simulink model "AGTF30SysDyn_PExPIn"  (R2021b)
settings: Solver=ode4  StartTime=0.0  StopTime=MWS.In.tend  FixedStep=MWS.In.Ts  RelTol=1e-3  EnableMultiTasking=on
model workspace: external: MAT-File (data not in the file)
values from neighbouring files (symbols this model uses):
  MWS = setup_initialize(MWS,startPt,SSsolverSP)    [Setup_Simulation.m]    (also in run_AGTF30e_script.m = Setup_Simulation(inputMethod,MWS.In,filename,Mdl,SSsolverSP,)
undefined symbols (not defined in the file or in its folder): DiscIntNeverNeededParam
libraries: Lib_Solve_ModelSource_TMATS x28, Lib_Cntrl_FirstOrderSensor_TMATS x19, simulink x12, Lib_Cntrl_FirstOrderActuator_TMATS x2, Lib_Cntrl_LimitSelect_TMATS x2, Lib_Solve_OuterLoopIntegrator_TMATS x2, Lib_Cntrl_CorrectedSpeed_TMATS x1, Lib_Solve_IterNRSolverJC_TMATS x1
(part 3 of 6)

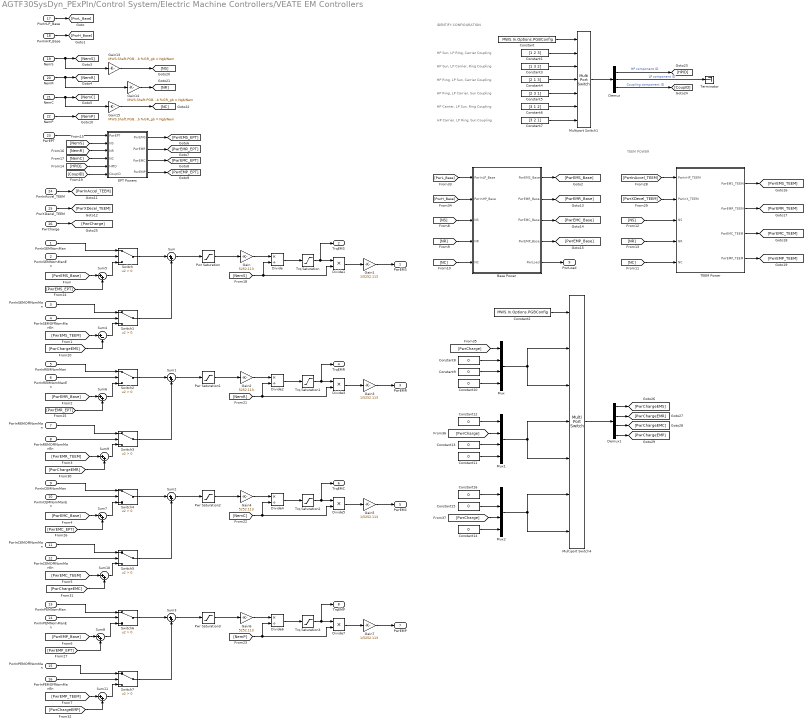
== system AGTF30SysDyn_PExPIn/Control System/Electric Machine Controllers/VEATE EM Controllers ==
  note: HP Sun, LP RIng, Carrier Coupling
  note: HP Sun, LP Carrier, Ring Coupling
  note: IDENTIFY CONFIGURATION
  note: HP Ring, LP Sun, Carrier Coupling
  note: HP Carrier, LP Sun, Ring Coupling
  note: HP Ring, LP Carrier, Sun Coupling
  note: HP Carrier, LP Ring, Sun Coupling
  note: TEEM POWER
  PwrInSEMNomMan : Inport
  PwrInSEMNomManEn : Inport  Port=2
  PwrInSEMOffNomMan : Inport  Port=3
  PwrInSEMOffNomManEn : Inport  Port=4
  PwrInREMNomMan : Inport  Port=5
  PwrInREMNomManEn : Inport  Port=6
  PwrInREMOffNomMan : Inport  Port=7
  PwrInREMOffNomManEn : Inport  Port=8
  PwrInCEMNomMan : Inport  Port=9
  PwrInCEMNomManEn : Inport  Port=10
  PwrInCEMOffNomMan : Inport  Port=11
  PwrInCEMOffNomManEn : Inport  Port=12
  PwrInPEMNomMan : Inport  Port=13
  PwrInPEMNomManEn : Inport  Port=14
  PwrInPEMOffNomMan : Inport  Port=15
  PwrInPEMOffNomManEn : Inport  Port=16
  PwrInLP_Base : Inport  Port=17
  PwrInHP_Base : Inport  Port=18
  NemS : Inport  Port=19
  NemR : Inport  Port=20
  NemC : Inport  Port=21
  NemP : Inport  Port=22
  PwrEPT : Inport  Port=23
  PwrInAccel_TEEM : Inport  Port=24
  PwrXDecel_TEEM : Inport  Port=25
  PwrCharge : Inport  Port=26
  Base Power : Subsystem
  Constant : Constant  Value=MWS.In.Options.PGBConfig
  Constant1 : Constant  Value=[1 2 3]
  Constant{8..16} (9 alike) : Constant  Value=0
  Constant2 : Constant  Value=MWS.In.Options.PGBConfig
  Constant3 : Constant  Value=[1 3 2]
  Constant4 : Constant  Value=[2 1 3]
  Constant5 : Constant  Value=[2 3 1]
  Constant6 : Constant  Value=[3 1 2]
  Constant7 : Constant  Value=[3 2 1]
  Demux : Demux  Outputs=3
  Demux1 : Demux
  Divide{,2,4,6} (4 alike) : Product  Inputs=*/
  Divide{1,3,5,7} (4 alike) : Product  Inputs=**
  EPT Powers : Subsystem
  Gain{,2,4,6} (4 alike) : Gain  Gain=5252.113
  Gain{1,3,5,7} (4 alike) : Gain  Gain=1/5252.113
  Gain13 : Gain  Gain=MWS.Shaft.PGB.Sun.GR_gb %GR_gb = Ngb/Nem
  Gain14 : Gain  Gain=MWS.Shaft.PGB.Ring.GR_gb %GR_gb = Ngb/Nem
  Gain15 : Gain  Gain=MWS.Shaft.PGB.Carrier.GR_gb %GR_gb = Ngb/Nem
  Multiport Switch1 : MultiPortSwitch  Inputs=6
  Multiport Switch4 : MultiPortSwitch  Inputs=6
  Mux : Mux
  Mux1 : Mux
  Mux2 : Mux
  Pwr Saturation : Saturate  UpperLimit=MWS.PowerSystem.EMS.PMax  LowerLimit=-MWS.PowerSystem.EMS.PMax
  Pwr Saturation1 : Saturate  UpperLimit=MWS.PowerSystem.EMR.PMax  LowerLimit=-MWS.PowerSystem.EMR.PMax
  Pwr Saturation2 : Saturate  UpperLimit=MWS.PowerSystem.EMC.PMax  LowerLimit=-MWS.PowerSystem.EMC.PMax
  Pwr Saturation3 : Saturate  UpperLimit=MWS.PowerSystem.EMP.PMax  LowerLimit=-MWS.PowerSystem.EMP.PMax
  Sum{,1..3,5..11} (11 alike) : Sum  Inputs=|++
  Sum4 : Sum  Inputs=|+-
  Switch{,1..7} (8 alike) : Switch  Criteria=u2 > Threshold
  TEEM Power : Subsystem
  Terminator : Terminator
  Trq Saturation : Saturate  UpperLimit=MWS.PowerSystem.EMS.TrqMax  LowerLimit=-MWS.PowerSystem.EMS.TrqMax
  Trq Saturation1 : Saturate  UpperLimit=MWS.PowerSystem.EMR.TrqMax  LowerLimit=-MWS.PowerSystem.EMR.TrqMax
  Trq Saturation2 : Saturate  UpperLimit=MWS.PowerSystem.EMC.TrqMax  LowerLimit=-MWS.PowerSystem.EMC.TrqMax
  Trq Saturation3 : Saturate  UpperLimit=MWS.PowerSystem.EMP.TrqMax  LowerLimit=-MWS.PowerSystem.EMP.TrqMax
  PwrEMS : Outport
  TrqEMS : Outport  Port=2
  PwrEMR : Outport  Port=3
  TrqEMR : Outport  Port=4
  PwrEMC : Outport  Port=5
  TrqEMC : Outport  Port=6
  PwrEMP : Outport  Port=7
  TrqEMP : Outport  Port=8
  PwrLoad : Outport  Port=9
  wires:
  PwrInSEMNomManEn/1 -> Switch/2
  PwrInSEMNomMan/1 -> Switch/1
  Switch/1 -> Sum/1
  Switch1/1 -> Sum/2
  PwrInSEMOffNomManEn/1 -> Switch1/2
  PwrInSEMOffNomMan/1 -> Switch1/1
  Sum/1 -> Pwr Saturation/1
  Pwr Saturation/1 -> Gain/1
  Gain/1 -> Divide/1
  [NemS] -> Divide/2, Divide1/2
  Divide/1 -> Trq Saturation/1
  Trq Saturation/1 -> Divide1/1, TrqEMS/1
  Divide1/1 -> Gain1/1
  Gain1/1 -> PwrEMS/1
  PwrInAccel_TEEM/1 -> [PwrInAccel_TEEM]
  PwrInLP_Base/1 -> [PwrL_Base]
  PwrInHP_Base/1 -> [PwrH_Base]
  [PwrEMS_Base] -> Sum5/1
  [PwrEMS_TEEM] -> Sum4/1
  Sum1/1 -> Pwr Saturation1/1
  Switch3/1 -> Sum1/2
  PwrInREMOffNomManEn/1 -> Switch3/2
  [PwrEMR_TEEM] -> Sum9/1
  [PwrEMR_Base] -> Sum6/1
  Divide3/1 -> Gain3/1
  [NemR] -> Divide2/2, Divide3/2
  Pwr Saturation1/1 -> Gain2/1
  Gain2/1 -> Divide2/1
  PwrInREMNomMan/1 -> Switch2/1
  Switch2/1 -> Sum1/1
  Divide2/1 -> Trq Saturation1/1
  Gain3/1 -> PwrEMR/1
  PwrInREMOffNomMan/1 -> Switch3/1
  Trq Saturation1/1 -> TrqEMR/1, Divide3/1
  PwrInREMNomManEn/1 -> Switch2/2
  Sum2/1 -> Pwr Saturation2/1
  Switch5/1 -> Sum2/2
  PwrInCEMOffNomManEn/1 -> Switch5/2
  [PwrEMC_TEEM] -> Sum10/1
  [PwrEMC_Base] -> Sum7/1
  Divide5/1 -> Gain5/1
  [NemC] -> Divide5/2, Divide4/2
  Pwr Saturation2/1 -> Gain4/1
  Gain4/1 -> Divide4/1
  PwrInCEMNomMan/1 -> Switch4/1
  Switch4/1 -> Sum2/1
  Divide4/1 -> Trq Saturation2/1
  Gain5/1 -> PwrEMC/1
  PwrInCEMOffNomMan/1 -> Switch5/1
  Trq Saturation2/1 -> TrqEMC/1, Divide5/1
  PwrInCEMNomManEn/1 -> Switch4/2
  Sum3/1 -> Pwr Saturation3/1
  Switch7/1 -> Sum3/2
  PwrInPEMOffNomManEn/1 -> Switch7/2
  [PwrEMP_TEEM] -> Sum11/1
  [PwrEMP_Base] -> Sum8/1
  Divide7/1 -> Gain7/1
  [NemP] -> Divide7/2, Divide6/2
  Pwr Saturation3/1 -> Gain6/1
  Gain6/1 -> Divide6/1
  PwrInPEMNomMan/1 -> Switch6/1
  Switch6/1 -> Sum3/1
  Divide6/1 -> Trq Saturation3/1
  Gain7/1 -> PwrEMP/1
  PwrInPEMOffNomMan/1 -> Switch7/1
  Trq Saturation3/1 -> TrqEMP/1, Divide7/1
  PwrInPEMNomManEn/1 -> Switch6/2
  NemS/1 -> Gain13/1, [NemS]
  NemC/1 -> Gain15/1, [NemC]
  NemP/1 -> [NemP]
  [NemC] -> EPT Powers/4(NC)
  [NemR] -> EPT Powers/3(NR)
  [NemS] -> EPT Powers/2(NS)
  PwrEPT/1 -> EPT Powers/1(PwrEPT)
  EPT Powers/1(PwrEMS) -> [PwrEMS_EPT]
  EPT Powers/2(PwrEMR) -> [PwrEMR_EPT]
  EPT Powers/3(PwrEMC) -> [PwrEMC_EPT]
  EPT Powers/4(PwrEMP) -> [PwrEMP_EPT]
  PwrXDecel_TEEM/1 -> [PwrXDecel_TEEM]
  Sum5/1 -> Switch/3
  [PwrEMS_EPT] -> Sum5/2
  Sum6/1 -> Switch2/3
  Sum7/1 -> Switch4/3
  Sum8/1 -> Switch6/3
  [PwrEMR_EPT] -> Sum6/2
  [PwrEMC_EPT] -> Sum7/2
  [PwrEMP_EPT] -> Sum8/2
  Gain13/1 -> [NS]
  Gain15/1 -> [NC]
  NemR/1 -> Gain14/1, [NemR]
  Gain14/1 -> [NR]
  Base Power/1(PwrEMS_Base) -> [PwrEMS_Base]
  Base Power/2(PwrEMR_Base) -> [PwrEMR_Base]
  Base Power/3(PwrEMC_Base) -> [PwrEMC_Base]
  Base Power/4(PwrEMP_Base) -> [PwrEMP_Base]
  [NC] -> Base Power/5(NC)
  [NR] -> Base Power/4(NR)
  [NS] -> Base Power/3(NS)
  [PwrH_Base] -> Base Power/2(PwrInHP_Base)
  [PwrL_Base] -> Base Power/1(PwrInLP_Base)
  [PwrInAccel_TEEM] -> TEEM Power/1(PwrInHP_TEEM)
  [PwrXDecel_TEEM] -> TEEM Power/2(PwrInX_TEEM)
  [NS] -> TEEM Power/3(NS)
  [NR] -> TEEM Power/4(NR)
  [NC] -> TEEM Power/5(NC)
  TEEM Power/1(PwrEMS_TEEM) -> [PwrEMS_TEEM]
  TEEM Power/2(PwrEMR_TEEM) -> [PwrEMR_TEEM]
  TEEM Power/3(PwrEMC_TEEM) -> [PwrEMC_TEEM]
  TEEM Power/4(PwrEMP_TEEM) -> [PwrEMP_TEEM]
  Demux/3 -> [CoupID]  "Coupling component ID"
  Demux/2 -> Terminator/1  "LP component ID"
  Constant5/1 -> Multiport Switch1/5
  Constant6/1 -> Multiport Switch1/6
  Multiport Switch1/1 -> Demux/1
  Constant1/1 -> Multiport Switch1/2
  Constant7/1 -> Multiport Switch1/7
  Constant/1 -> Multiport Switch1/1
  Constant3/1 -> Multiport Switch1/3
  Constant4/1 -> Multiport Switch1/4
  Demux/1 -> [HPID]  "HP component ID"
  [HPID] -> EPT Powers/5(HPID)
  [CoupID] -> EPT Powers/6(CoupID)
  PwrCharge/1 -> [PwrCharge]
  Base Power/5(PwrLoad) -> PwrLoad/1
  Sum4/1 -> Switch1/3
  [PwrChargeEMS] -> Sum4/2
  [PwrChargeEMR] -> Sum9/2
  [PwrChargeEMC] -> Sum10/2
  [PwrChargeEMP] -> Sum11/2
  Sum9/1 -> Switch3/3
  Sum10/1 -> Switch5/3
  Sum11/1 -> Switch7/3
  Constant2/1 -> Multiport Switch4/1
  Multiport Switch4/1 -> Demux1/1
  [PwrCharge] -> Mux/1
  Constant8/1 -> Mux/2
  Constant9/1 -> Mux/3
  Constant10/1 -> Mux/4
  Demux1/1 -> [PwrChargeEMS]
  Demux1/2 -> [PwrChargeEMR]
  Demux1/3 -> [PwrChargeEMC]
  Demux1/4 -> [PwrChargeEMP]
  Mux/1 -> Multiport Switch4/2, Multiport Switch4/3
  Constant11/1 -> Mux1/4
  [PwrCharge] -> Mux1/2
  Constant12/1 -> Mux1/1
  Constant13/1 -> Mux1/3
  Mux1/1 -> Multiport Switch4/5, Multiport Switch4/4
  Constant14/1 -> Mux2/4
  [PwrCharge] -> Mux2/3
  Constant15/1 -> Mux2/2
  Constant16/1 -> Mux2/1
  Mux2/1 -> Multiport Switch4/6, Multiport Switch4/7

== system AGTF30SysDyn_PExPIn/Control System/Scheduling/MaxMin Fuel Flow Calc ==
  k_Alt : Inport
  f_Alt : Inport  Port=2
  k_MN : Inport  Port=3
  f_MN : Inport  Port=4
  k_PwrInLPMx : Inport  Port=5
  f_PwrInLPMx : Inport  Port=6
  k_PwrInLPMn : Inport  Port=7
  f_PwrInLPMn : Inport  Port=8
  k_PwrInHPMx : Inport  Port=9
  f_PwrInHPMx : Inport  Port=10
  k_PwrInHPMn : Inport  Port=11
  f_PwrInHPMn : Inport  Port=12
  Wfmax Interpolation Using Prelookup : Interpolation_n-D  NumberOfTableDimensions=4  Table=MWS.Cntrl.Sched.WfMax.WfMax_array  InternalRulePriority=Speed
      settings: InputPortMap=u0,u1,u2,u3,u4,u5,u6,u7
  Wfmin Interpolation Using Prelookup : Interpolation_n-D  NumberOfTableDimensions=4  Table=MWS.Cntrl.Sched.WfMin.WfMin_array  InternalRulePriority=Speed
      settings: InputPortMap=u0,u1,u2,u3,u4,u5,u6,u7
  Wfmin : Outport  VectorParamsAs1DForOutWhenUnconnected=off
  Wfmax : Outport  Port=2  VectorParamsAs1DForOutWhenUnconnected=off
  wires:
  f_PwrInLPMn/1 -> Wfmin Interpolation Using Prelookup/6
  k_PwrInLPMn/1 -> Wfmin Interpolation Using Prelookup/5
  f_PwrInLPMx/1 -> Wfmax Interpolation Using Prelookup/6
  k_PwrInLPMx/1 -> Wfmax Interpolation Using Prelookup/5
  f_MN/1 -> Wfmax Interpolation Using Prelookup/4, Wfmin Interpolation Using Prelookup/4
  k_MN/1 -> Wfmax Interpolation Using Prelookup/3, Wfmin Interpolation Using Prelookup/3
  f_Alt/1 -> Wfmax Interpolation Using Prelookup/2, Wfmin Interpolation Using Prelookup/2
  k_Alt/1 -> Wfmax Interpolation Using Prelookup/1, Wfmin Interpolation Using Prelookup/1
  Wfmin Interpolation Using Prelookup/1 -> Wfmin/1
  Wfmax Interpolation Using Prelookup/1 -> Wfmax/1
  k_PwrInHPMx/1 -> Wfmax Interpolation Using Prelookup/7
  f_PwrInHPMx/1 -> Wfmax Interpolation Using Prelookup/8
  k_PwrInHPMn/1 -> Wfmin Interpolation Using Prelookup/7
  f_PwrInHPMn/1 -> Wfmin Interpolation Using Prelookup/8

== system AGTF30SysDyn_PExPIn/Control System/Scheduling/Power Level Lookup Determination ==
  k_Alt : Inport
  f_Alt : Inport  Port=2
  k_MN : Inport  Port=3
  f_MN : Inport  Port=4
  k_PwrInLPMn : Inport  Port=5
  f_PwrInLPMx : Inport  Port=6
  k_PwrInHPMn : Inport  Port=7
  f_PwrInHPMx : Inport  Port=8
  FnTarget : Inport  Port=9
  N1c : Inport  Port=10
  Constant1 : Constant  Value=MWS.Cntrl.SPSched.PL_vec
  Constant35 : Constant  Value=[[0:1:length(MWS.Cntrl.SPSched.PL_vec)-2],length(MWS.Cntrl.SPSched.PL_vec)-2]
  Constant36 : Constant  Value=[zeros(1,length(MWS.Cntrl.SPSched.PL_vec)-1),1]
  Fn Interpolation Using Prelookup : Interpolation_n-D  NumberOfTableDimensions=5  Table=MWS.Cntrl.Sched.Fn.Fn_array  InternalRulePriority=Speed
      settings: InputPortMap=u0,u1,u2,u3,u4,u5,u6,u7,u8,u9
  Fn Lookup Table Dynamic : simulink/Lookup Tables/Lookup Table Dynamic  LookUpMeth=Interpolation-Use End Values  OutDataType=fixdt('double')  OutScaling=[]  OutputDataTypeScalingMode=Specify via dialog  OutDataTypeStr=double  DoSatur=off
  N1c Interpolation Using Prelookup1 : Interpolation_n-D  NumberOfTableDimensions=5  Table=MWS.Cntrl.WfCntrl.Sched.N1cSP.N1cSP_array  InternalRulePriority=Speed
      settings: InputPortMap=u0,u1,u2,u3,u4,u5,u6,u7,u8,u9
  N1c Lookup Table Dynamic : simulink/Lookup Tables/Lookup Table Dynamic  LookUpMeth=Interpolation-Use End Values  OutDataType=fixdt('double')  OutScaling=[]  OutputDataTypeScalingMode=Specify via dialog  OutDataTypeStr=double  DoSatur=off
  PL Prelookup1 : PreLookup  BreakpointsData=MWS.Cntrl.SPSched.PL_vec  IndexSearchMethod=Linear search  BeginIndexSearchUsingPreviousIndexResult=on  ExtrapMethod=Linear
  PL Targ Prelookup : PreLookup  BreakpointsData=MWS.Cntrl.SPSched.PL_vec  IndexSearchMethod=Linear search  BeginIndexSearchUsingPreviousIndexResult=on  ExtrapMethod=Linear
  k_PL_Targ : Outport
  f_PL_Targ : Outport  Port=2
  k_PL : Outport  Port=3
  f_PL : Outport  Port=4
  wires:
  f_PwrInHPMx/1 -> N1c Interpolation Using Prelookup1/10, Fn Interpolation Using Prelookup/10
  f_PwrInLPMx/1 -> N1c Interpolation Using Prelookup1/8, Fn Interpolation Using Prelookup/8
  k_PwrInHPMn/1 -> N1c Interpolation Using Prelookup1/9, Fn Interpolation Using Prelookup/9
  k_Alt/1 -> N1c Interpolation Using Prelookup1/3, Fn Interpolation Using Prelookup/3
  f_MN/1 -> N1c Interpolation Using Prelookup1/6, Fn Interpolation Using Prelookup/6
  k_MN/1 -> N1c Interpolation Using Prelookup1/5, Fn Interpolation Using Prelookup/5
  Constant35/1 -> N1c Interpolation Using Prelookup1/1, Fn Interpolation Using Prelookup/1
  f_Alt/1 -> N1c Interpolation Using Prelookup1/4, Fn Interpolation Using Prelookup/4
  k_PwrInLPMn/1 -> N1c Interpolation Using Prelookup1/7, Fn Interpolation Using Prelookup/7
  Constant36/1 -> N1c Interpolation Using Prelookup1/2, Fn Interpolation Using Prelookup/2
  Fn Interpolation Using Prelookup/1 -> [FnVec]
  FnTarget/1 -> Fn Lookup Table Dynamic/1
  [FnVec] -> Fn Lookup Table Dynamic/2
  Constant1/1 -> N1c Lookup Table Dynamic/3, Fn Lookup Table Dynamic/3
  Fn Lookup Table Dynamic/1 -> PL Targ Prelookup/1  "PL"
  PL Targ Prelookup/2 -> f_PL_Targ/1  "f_PL_Fn"
  PL Targ Prelookup/1 -> k_PL_Targ/1  "k_PL_Fn"
  N1c Lookup Table Dynamic/1 -> PL Prelookup1/1  "PL"
  PL Prelookup1/2 -> f_PL/1  "f_PL_Fn"
  PL Prelookup1/1 -> k_PL/1  "k_PL_Fn"
  [N1cVec] -> N1c Lookup Table Dynamic/2
  N1c Interpolation Using Prelookup1/1 -> [N1cVec]
  N1c/1 -> N1c Lookup Table Dynamic/1

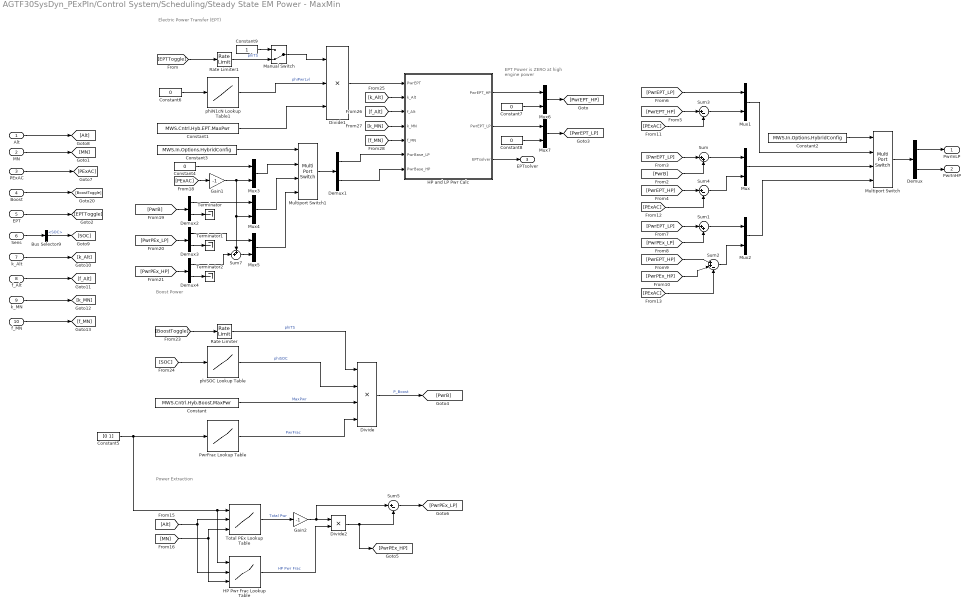
== system AGTF30SysDyn_PExPIn/Control System/Scheduling/Steady State EM Power - MaxMin ==
  note: EPT Power is ZERO at high engine power
  note: Electric Power Transfer (EPT)
  note: Boost Power
  note: Power Extraction
  Alt : Inport
  MN : Inport  Port=2
  PExAC : Inport  Port=3
  Boost : Inport  Port=4
  EPT : Inport  Port=5
  Sens : Inport  Port=6
  k_Alt : Inport  Port=7
  f_Alt : Inport  Port=8
  k_MN : Inport  Port=9
  f_MN : Inport  Port=10
  Bus Selector9 : BusSelector  OutputSignals=SOC
  Constant : Constant  Value=MWS.Cntrl.Hyb.Boost.MaxPwr
  Constant1 : Constant  Value=MWS.Cntrl.Hyb.EPT.MaxPwr
  Constant2 : Constant  Value=MWS.In.Options.HybridConfig
  Constant3 : Constant  Value=MWS.In.Options.HybridConfig
  Constant{4,6..8} (4 alike) : Constant  Value=0
  Constant5 : Constant  Value=[0 1]
  Constant9 : Constant
  Demux{,1..4} (5 alike) : Demux  Outputs=2
  Divide : Product  Inputs=****
  Divide1 : Product  Inputs=***
  Divide2 : Product  Inputs=**
  Gain1 : Gain  Gain=-1
  Gain2 : Gain  Gain=-1
  HP Pwr Frac Lookup Table : Lookup_n-D  NumberOfTableDimensions=3  BreakpointsForDimension1=MWS.Cntrl.Hyb.PEx.PwrSplitSched.NcFanN_vec  BreakpointsForDimension2=MWS.Cntrl.Hyb.PEx.PwrSplitSched.Alt_vec  BreakpointsForDimension3=MWS.Cntrl.Hyb.PEx.PwrSplitSched.MN_vec  Table=MWS.Cntrl.Hyb.PEx.PwrSplitSched.PwrFracHP_array  InternalRulePriority=Speed  RndMeth=Simplest  InputSameDT=on
      settings: InputPortMap=u0,u1,u2
  HP and LP Pwr Calc : Subsystem
  Manual Switch : ManualSwitch  CurrentSetting=0
  Multiport Switch : MultiPortSwitch
  Multiport Switch1 : MultiPortSwitch
  Mux{,1..7} (8 alike) : Mux  Inputs=2
  PwrFrac Lookup Table : Lookup_n-D  NumberOfTableDimensions=1  BreakpointsForDimension1=MWS.Cntrl.Hyb.Boost.PwrFracSched.NcFanN_vec  BreakpointsForDimension2=MWS.Cntrl.PHpwr.Sched.MN_vec  Table=MWS.Cntrl.Hyb.Boost.PwrFracSched.PwrFrac_vec  InternalRulePriority=Speed  RndMeth=Simplest  InputSameDT=on
  Rate Limiter : RateLimiter  RisingSlewLimit=MWS.Cntrl.Hyb.Boost.RL  FallingSlewLimit=-MWS.Cntrl.Hyb.Boost.RL  SampleTimeMode=inherited
  Rate Limiter1 : RateLimiter  RisingSlewLimit=MWS.Cntrl.Hyb.EPT.RL  FallingSlewLimit=-MWS.Cntrl.Hyb.EPT.RL  SampleTimeMode=inherited
  Sum : Sum  Inputs=|++
  Sum1 : Sum  Inputs=|++
  Sum2 : Sum  Inputs=|++-
  Sum3 : Sum  Inputs=|+-
  Sum4 : Sum  Inputs=|+-
  Sum5 : Sum  Inputs=|+-
  Sum7 : Sum  Inputs=++|
  Terminator : Terminator
  Terminator1 : Terminator
  Terminator2 : Terminator
  Total PEx Lookup Table : Lookup_n-D  NumberOfTableDimensions=3  BreakpointsForDimension1=MWS.Cntrl.Hyb.PEx.PExSched.NcFanN_vec  BreakpointsForDimension2=MWS.Cntrl.Hyb.PEx.PExSched.Alt_vec  BreakpointsForDimension3=MWS.Cntrl.Hyb.PEx.PExSched.MN_vec  Table=MWS.Cntrl.Hyb.PEx.PExSched.Pwr_array  InternalRulePriority=Speed  RndMeth=Simplest  InputSameDT=on
      settings: InputPortMap=u0,u1,u2
  phiN1cN Lookup Table1 : Lookup_n-D  NumberOfTableDimensions=1  BreakpointsForDimension1=MWS.Cntrl.Hyb.EPT.Sched.N1cN_vec  BreakpointsForDimension2=MWS.Cntrl.PHpwr.Sched.MN_vec  Table=MWS.Cntrl.Hyb.EPT.Sched.phiPwrLvl_vec  InternalRulePriority=Speed  RndMeth=Simplest  InputSameDT=on
  phiSOC Lookup Table : Lookup_n-D  NumberOfTableDimensions=1  BreakpointsForDimension1=MWS.Cntrl.Hyb.Boost.phiSOCSched.SOC_vec  BreakpointsForDimension2=MWS.Cntrl.PHpwr.Sched.MN_vec  Table=MWS.Cntrl.Hyb.Boost.phiSOCSched.phiSOC_vec  InternalRulePriority=Speed  RndMeth=Simplest  InputSameDT=on
  PwrInLP : Outport
  PwrInHP : Outport  Port=2
  EPTsolver : Outport  Port=3
  wires:
  Constant/1 -> Divide/3  "MaxPwr"
  MN/1 -> [MN]
  [SOC] -> phiSOC Lookup Table/1
  phiSOC Lookup Table/1 -> Divide/2  "phiSOC"
  [BoostToggle] -> Rate Limiter/1
  Alt/1 -> [Alt]
  PwrFrac Lookup Table/1 -> Divide/4  "PwrFrac"
  Sens/1 -> Bus Selector9/1
  Rate Limiter/1 -> Divide/1  "phiTS"
  Boost/1 -> [BoostToggle]
  Divide/1 -> [PwrB]  "P_Boost"
  [EPTToggle] -> Rate Limiter1/1
  Constant6/1 -> phiN1cN Lookup Table1/1
  phiN1cN Lookup Table1/1 -> Divide1/2  "phiPwrLvl"
  Rate Limiter1/1 -> Manual Switch/2  "phiTS"
  [PwrEPT_LP] -> Sum/1
  [PwrB] -> Sum/2
  [PwrEPT_LP] -> Mux1/1
  Sum/1 -> Mux/1
  [PwrEPT_HP] -> Sum4/1
  [PwrEPT_LP] -> Sum1/1
  [PwrPEx_LP] -> Sum1/2
  [PwrEPT_HP] -> Sum2/1
  [PwrPEx_HP] -> Sum2/2
  Sum2/1 -> Mux2/2
  Sum1/1 -> Mux2/1
  Mux1/1 -> Multiport Switch/2
  Mux/1 -> Multiport Switch/3
  Mux2/1 -> Multiport Switch/4
  Constant2/1 -> Multiport Switch/1
  [PwrEPT_HP] -> Sum3/1
  [PExAC] -> Sum3/2
  Sum3/1 -> Mux1/2
  Multiport Switch/1 -> Demux/1
  Demux/1 -> PwrInLP/1
  Demux/2 -> PwrInHP/1
  [PExAC] -> Sum4/2
  [PExAC] -> Sum2/3
  Sum4/1 -> Mux/2
  Constant5/1 -> HP Pwr Frac Lookup Table/1, Total PEx Lookup Table/1, PwrFrac Lookup Table/1
  [Alt] -> HP Pwr Frac Lookup Table/2, Total PEx Lookup Table/2
  [MN] -> HP Pwr Frac Lookup Table/3, Total PEx Lookup Table/3
  Total PEx Lookup Table/1 -> Gain2/1  "Total Pwr"
  HP Pwr Frac Lookup Table/1 -> Divide2/2  "HP Pwr Frac"
  Divide2/1 -> [PwrPEx_HP], Sum5/2
  Gain2/1 -> Divide2/1, Sum5/1
  Sum5/1 -> [PwrPEx_LP]
  EPT/1 -> [EPTToggle]
  PExAC/1 -> [PExAC]
  Constant1/1 -> Divide1/3
  Bus Selector9/1 -> [SOC]  "<SOC>"
  Constant3/1 -> Multiport Switch1/1
  Constant4/1 -> Mux3/1
  [PExAC] -> Gain1/1
  Mux3/1 -> Multiport Switch1/2
  Gain1/1 -> Mux3/2, Mux4/2, Sum7/1
  Sum7/1 -> Mux5/2
  Mux4/1 -> Multiport Switch1/3
  Mux5/1 -> Multiport Switch1/4
  Multiport Switch1/1 -> Demux1/1
  Demux1/1 -> HP and LP Pwr Calc/6(PwrBase_LP)
  Demux1/2 -> HP and LP Pwr Calc/7(PwrBase_HP)
  k_Alt/1 -> [k_Alt]
  f_Alt/1 -> [f_Alt]
  k_MN/1 -> [k_MN]
  f_MN/1 -> [f_MN]
  [f_Alt] -> HP and LP Pwr Calc/3(f_Alt)
  [k_MN] -> HP and LP Pwr Calc/4(k_MN)
  [f_MN] -> HP and LP Pwr Calc/5(f_MN)
  [k_Alt] -> HP and LP Pwr Calc/2(k_Alt)
  Divide1/1 -> HP and LP Pwr Calc/1(PwrEPT)
  HP and LP Pwr Calc/3(EPTsolver) -> EPTsolver/1
  Mux6/1 -> [PwrEPT_HP]
  Mux7/1 -> [PwrEPT_LP]
  HP and LP Pwr Calc/1(PwrEPT_HP) -> Mux6/1
  HP and LP Pwr Calc/2(PwrEPT_LP) -> Mux7/1
  Constant7/1 -> Mux6/2
  Constant8/1 -> Mux7/2
  Demux2/2 -> Terminator/1
  [PwrB] -> Demux2/1
  Demux2/1 -> Mux4/1
  [PwrPEx_LP] -> Demux3/1
  [PwrPEx_HP] -> Demux4/1
  Demux3/2 -> Terminator1/1
  Demux4/2 -> Terminator2/1
  Demux4/1 -> Sum7/2
  Demux3/1 -> Mux5/1
  Constant9/1 -> Manual Switch/1
  Manual Switch/1 -> Divide1/1

== system AGTF30SysDyn_PExPIn/Control System/Wf Controller/Controller ==
  Prelookup : Inport
  Alt : Inport  Port=2
  MN : Inport  Port=3
  N1c : Inport  Port=4
  N1 : Inport  Port=5
  N3 : Inport  Port=6
  Ps3 : Inport  Port=7
  T3 : Inport  Port=8
  T4 : Inport  Port=9
  T45 : Inport  Port=10
  NcFanManEn : Inport  Port=11
  NcFanMan : Inport  Port=12
  Wfmin : Inport  Port=13
  Wfmax : Inport  Port=14
  phiEPT : Inport  Port=15
  phiBoost : Inport  Port=16
  N1cN : Inport  Port=17
  Bus Creator : BusCreator  Inputs=2
  Mux1 : Mux  Inputs=7
  Mux2 : Mux  Inputs=3
  N1cSP Limit Controllers : Subsystem
  N1cSP Limit Select : Subsystem
  Nominal Controller : Subsystem
  Nominal Set-Point Determination : Subsystem
  Set-Points : Subsystem
  Wf Limit Controllers : Subsystem
  Wf Limit Select : Subsystem
  Wfdmd : Outport  VectorParamsAs1DForOutWhenUnconnected=off
  RegNum : Outport  Port=2  VectorParamsAs1DForOutWhenUnconnected=off
  SPs : Outport  Port=3  VectorParamsAs1DForOutWhenUnconnected=off
  N1cErr : Outport  Port=4  VectorParamsAs1DForOutWhenUnconnected=off
  wires:
  N1c/1 -> Nominal Controller/5(N1c)
  Prelookup/1 -> [Prelookup], N1cSP Limit Controllers/1(Prelookup), Nominal Set-Point Determination/1(Prelookup)
  N1cSP Limit Select/1(N1cSPdmd) -> Nominal Controller/4(N1cSP), N1cSP Limit Controllers/8(N1cCmd)
  T4/1 -> N1cSP Limit Controllers/6(T4)
  N3/1 -> N1cSP Limit Controllers/3(N3)
  Ps3/1 -> Wf Limit Controllers/9(ps3), N1cSP Limit Controllers/4(Ps3)
  T3/1 -> N1cSP Limit Controllers/5(T3)
  Nominal Set-Point Determination/1(N1cSP) -> Set-Points/1(Nominal SP), N1cSP Limit Select/1(N1cSPReq)
  N1cSP Limit Controllers/8(SPs) -> Set-Points/2(N1cSP Limit SPs)
  Set-Points/1(SPs) -> SPs/1
  N1/1 -> N1cSP Limit Controllers/2(N1)
  N1cSP Limit Controllers/7(N1cSP Ps3 Min) -> Mux1/7
  N1cSP Limit Controllers/5(N1cSP N3 Max) -> Mux1/5
  N1cSP Limit Controllers/4(N1cSP N1 Max) -> Mux1/4
  N1cSP Limit Controllers/6(N1cSP Ps3 Max) -> Mux1/6
  N1cSP Limit Controllers/2(N1cSP T4 Max) -> Mux1/2
  NcFanManEn/1 -> Nominal Controller/2(N1cManEn)
  N1cSP Limit Controllers/1(N1cSP T3 Max) -> Mux1/1
  [Prelookup] -> Nominal Controller/1(Prelookup)
  Nominal Controller/1(Wfdmd) -> Wf Limit Select/1(WfReq)
  Wf Limit Select/1(Wfdmd) -> Nominal Controller/6(Wfcmd), Wf Limit Controllers/5(Wfcmd), Wfdmd/1
  Wfmin/1 -> Wf Limit Controllers/3(Wfmin)
  Wfmax/1 -> Wf Limit Controllers/4(Wfmax)
  Wf Limit Controllers/1(Wf Accel) -> Mux2/1
  Wf Limit Controllers/2(Wf Decel) -> Mux2/2
  Wf Limit Controllers/3(Wf Min) -> Mux2/3
  Mux2/1 -> Wf Limit Select/2(Limits)
  Wf Limit Controllers/4(SPs) -> Set-Points/3(Wf Limit SPs)
  Alt/1 -> Wf Limit Controllers/1(Alt)
  T45/1 -> N1cSP Limit Controllers/7(T45)
  N1cSP Limit Controllers/3(N1cSP T45 Max) -> Mux1/3
  NcFanMan/1 -> Nominal Controller/3(N1cMan)
  Bus Creator/1 -> RegNum/1
  N1cSP Limit Select/2(RegNum) -> Bus Creator/1  "N1cSP"
  Wf Limit Select/2(RegNum) -> Bus Creator/2  "Wf"
  Nominal Controller/2(N1cErr) -> N1cErr/1
  Mux1/1 -> N1cSP Limit Select/2(Limits)
  MN/1 -> Wf Limit Controllers/2(MN)
  phiEPT/1 -> Wf Limit Controllers/6(phiEPT)
  phiBoost/1 -> Wf Limit Controllers/7(phiBoost)
  N1cN/1 -> Wf Limit Controllers/8(N1cN)

== system AGTF30SysDyn_PExPIn/Control System/Wf Controller/Corrected Speed Calc ==
  N : Inport
  T : Inport  Port=2
  Divide : Product  Inputs=*/
  Gain : Gain  Gain=1/518.67
  Sqrt : Sqrt  SaturateOnIntegerOverflow=on
  Nc : Outport  VectorParamsAs1DForOutWhenUnconnected=off
  wires:
  Sqrt/1 -> Divide/2
  N/1 -> Divide/1
  T/1 -> Gain/1
  Gain/1 -> Sqrt/1
  Divide/1 -> Nc/1

== system AGTF30SysDyn_PExPIn/EngineSystem/EngineDW/Subsystem ==
  SysIn : Inport
  N : Inport  Port=2
  Bus Selector4 : BusSelector  OutputSignals=CntrlInp.ManualOp.PwrInLPNomMan,CntrlInp.ManualOp.PwrInLPNomManEn,CntrlInp.ManualOp.PwrInLPOffNomMan,CntrlInp.ManualOp.PwrInLPOffNomManEn,CntrlInp.ManualOp.PwrInHPNomMan,CntrlInp.ManualOp.PwrInHPNomManEn,CntrlInp.ManualOp.PwrInHPOffNomMan,CntrlInp.ManualOp.PwrInHPOffNomManEn
  Constant{,1..3} (4 alike) : Constant  Value=0
  Demux : Demux  Outputs=2
  Divide : Product  Inputs=*/
  Divide1 : Product  Inputs=/*
  Gain : Gain  Gain=5252.113
  Gain1 : Gain  Gain=5252.113
  Sum : Sum  Inputs=|++
  Sum1 : Sum  Inputs=|++
  Switch{,1..3} (4 alike) : Switch  Criteria=u2 > Threshold
  TrqInLP : Outport
  TrqInHP : Outport  Port=2
  wires:
  SysIn/1 -> Bus Selector4/1
  Bus Selector4/1 -> [PwrLPNom]  "<PwrInLPNomMan>"
  Bus Selector4/2 -> [EnPwrLPNom]  "<PwrInLPNomManEn>"
  Bus Selector4/3 -> [PwrLPOffNom]  "<PwrInLPOffNomMan>"
  Bus Selector4/4 -> [EnPwrLPOffNom]  "<PwrInLPOffNomManEn>"
  [EnPwrLPNom] -> Switch/2
  Constant/1 -> Switch/3
  [PwrLPNom] -> Switch/1
  [PwrLPOffNom] -> Switch1/1
  Constant1/1 -> Switch1/3
  [EnPwrLPOffNom] -> Switch1/2
  Switch/1 -> Sum/1
  Switch1/1 -> Sum/2
  Sum/1 -> Divide/1
  Sum1/1 -> Divide1/2
  Switch3/1 -> Sum1/2
  Switch2/1 -> Sum1/1
  [EnPwrHPOffNom] -> Switch3/2
  Constant3/1 -> Switch3/3
  [PwrHPOffNom] -> Switch3/1
  [PwrHPNom] -> Switch2/1
  Constant2/1 -> Switch2/3
  [EnPwrHPNom] -> Switch2/2
  Bus Selector4/5 -> [PwrHPNom]  "<PwrInHPNomMan>"
  Bus Selector4/6 -> [EnPwrHPNom]  "<PwrInHPNomManEn>"
  Bus Selector4/7 -> [PwrHPOffNom]  "<PwrInHPOffNomMan>"
  Bus Selector4/8 -> [EnPwrHPOffNom]  "<PwrInHPOffNomManEn>"
  N/1 -> Demux/1
  Divide/1 -> Gain/1
  Gain/1 -> TrqInLP/1
  Divide1/1 -> Gain1/1
  Gain1/1 -> TrqInHP/1
  Demux/1 -> Divide/2
  Demux/2 -> Divide1/1

== system AGTF30SysDyn_PExPIn/EngineSystem/Power System/SOC Calc ==
  <Supplybranch> : Inport
  1 : Constant  Value=100
  Demux2 : Demux  Outputs=[3 1]
  Divide1 : Product  Inputs=*/
  "Energy Storage Capacity, kW-hr" : Constant  Value=MWS.PowerSystem.ESD.EnergyCapacity
  "Initial SOC, %" : Constant  Value=MWS.Init.IC.SOC
  Integrator : Integrator
  J to kW-hr : Gain  Gain=2.77778*10^-7
  Product1 : Product
  Saturation : Saturate  UpperLimit=100  LowerLimit=0
  Sum3 : Sum  Inputs=|-+
  Terminator : Terminator
  ESD SOC : Outport
  wires:
  Divide1/1 -> Product1/1
  "Initial SOC, %"/1 -> Sum3/2
  J to kW-hr/1 -> Divide1/1
  1/1 -> Product1/2
  Product1/1 -> Sum3/1
  Demux2/2 -> Integrator/1  "ESD Pwr"
  "Energy Storage Capacity, kW-hr"/1 -> Divide1/2
  Demux2/1 -> Terminator/1
  Integrator/1 -> J to kW-hr/1  "ESD Energy [J]"
  Sum3/1 -> Saturation/1  "ESD SOC"
  Saturation/1 -> ESD SOC/1  "ESD SOC"
  <Supplybranch>/1 -> Demux2/1

== system AGTF30SysDyn_PExPIn/Control System/Electric Machine Controllers/DEM EM Controllers/EMH Controller ==
  PwrInHPEMNomMan : Inport
  PwrInHPEMNomManEn : Inport  Port=2
  PwrInHPEMOffNomMan : Inport  Port=3
  PwrInHPEMOffNomManEn : Inport  Port=4
  PwrInHP_Base : Inport  Port=5
  NemH : Inport  Port=6
  PwrInHPEPT : Inport  Port=7
  PwrInAccel_TEEM : Inport  Port=8
  PwrXDecel_TEEM : Inport  Port=9
  PwrCharge : Inport  Port=10
  Divide : Product  Inputs=*/
  Divide1 : Product  Inputs=**
  Gain : Gain  Gain=5252.113
  Gain1 : Gain  Gain=1/5252.113
  Pwr Saturation : Saturate  UpperLimit=MWS.PowerSystem.EMH.PMax  LowerLimit=-MWS.PowerSystem.EMH.PMax
  Sum : Sum  Inputs=|++
  Sum1 : Sum  Inputs=|++
  Sum2 : Sum  Inputs=|++
  Sum3 : Sum  Inputs=|+-
  Switch : Switch  Criteria=u2 > Threshold
  Switch1 : Switch  Criteria=u2 > Threshold
  Trq Saturation : Saturate  UpperLimit=MWS.PowerSystem.EMH.TrqMax  LowerLimit=-MWS.PowerSystem.EMH.TrqMax
  PwrEMH : Outport
  TrqEMH : Outport  Port=2
  wires:
  Gain1/1 -> PwrEMH/1
  Divide1/1 -> Gain1/1
  Trq Saturation/1 -> Divide1/1, TrqEMH/1
  Divide/1 -> Trq Saturation/1
  NemH/1 -> Divide/2, Divide1/2
  Gain/1 -> Divide/1
  Pwr Saturation/1 -> Gain/1
  Sum/1 -> Pwr Saturation/1
  Sum1/1 -> Sum3/1  "Pwr_TEEM"
  PwrInHPEMOffNomMan/1 -> Switch1/1
  PwrInHPEMOffNomManEn/1 -> Switch1/2
  Switch1/1 -> Sum/2
  Switch/1 -> Sum/1
  PwrInHP_Base/1 -> Sum2/1
  PwrInHPEMNomMan/1 -> Switch/1
  PwrInHPEMNomManEn/1 -> Switch/2
  PwrXDecel_TEEM/1 -> Sum1/2
  Sum2/1 -> Switch/3  "PwrSS"
  PwrInHPEPT/1 -> Sum2/2
  Sum3/1 -> Switch1/3  "Pwr_OffNom"
  PwrCharge/1 -> Sum3/2
  PwrInAccel_TEEM/1 -> Sum1/1

== system AGTF30SysDyn_PExPIn/Control System/Electric Machine Controllers/DEM EM Controllers/EML Controller ==
  PwrInLPEMNomMan : Inport
  PwrInLPEMNomManEn : Inport  Port=2
  PwrInLPEMOffNomMan : Inport  Port=3
  PwrInLPEMOffNomManEn : Inport  Port=4
  PwrInLP_Base : Inport  Port=5
  NemL : Inport  Port=6
  PwrInLPEPT : Inport  Port=7
  PwrXDecel_TEEM : Inport  Port=8
  Divide : Product  Inputs=*/
  Divide1 : Product  Inputs=**
  Gain : Gain  Gain=5252.113
  Gain1 : Gain  Gain=1/5252.113
  Gain2 : Gain  Gain=-1
  Pwr Saturation : Saturate  UpperLimit=MWS.PowerSystem.EML.PMax  LowerLimit=-MWS.PowerSystem.EML.PMax
  Sum : Sum  Inputs=|++
  Sum1 : Sum  Inputs=|++
  Switch : Switch  Criteria=u2 > Threshold
  Switch1 : Switch  Criteria=u2 > Threshold
  Trq Saturation : Saturate  UpperLimit=MWS.PowerSystem.EML.TrqMax  LowerLimit=-MWS.PowerSystem.EML.TrqMax
  PwrEML : Outport
  TrqEML : Outport  Port=2
  wires:
  PwrInLPEMNomManEn/1 -> Switch/2
  PwrInLPEMNomMan/1 -> Switch/1
  PwrInLP_Base/1 -> Sum1/1
  Switch/1 -> Sum/1
  Switch1/1 -> Sum/2
  PwrInLPEMOffNomManEn/1 -> Switch1/2
  PwrInLPEMOffNomMan/1 -> Switch1/1
  Gain2/1 -> Switch1/3  "PwrInLPS_TEEM"
  Sum/1 -> Pwr Saturation/1
  Pwr Saturation/1 -> Gain/1
  Gain/1 -> Divide/1
  NemL/1 -> Divide1/2, Divide/2
  Divide/1 -> Trq Saturation/1
  Trq Saturation/1 -> TrqEML/1, Divide1/1
  Divide1/1 -> Gain1/1
  Gain1/1 -> PwrEML/1
  PwrXDecel_TEEM/1 -> Gain2/1
  PwrInLPEPT/1 -> Sum1/2
  Sum1/1 -> Switch/3

== system AGTF30SysDyn_PExPIn/Control System/Electric Machine Controllers/DEM EM Controllers/EPT Pwr Calc ==
  PwrEPT : Inport
  Gain : Gain  Gain=-1
  PwrEML_EPT : Outport
  PwrEMH_EPT : Outport  Port=2
  wires:
  Gain/1 -> PwrEML_EPT/1
  PwrEPT/1 -> PwrEMH_EPT/1, Gain/1

== system AGTF30SysDyn_PExPIn/Control System/Electric Machine Controllers/VEATE EM Controllers/Base Power ==
  note: STRATEGY WILL USE THE COUPLING EM AS MUCH AS POSSIBLE AND WILL FILL IN THE REST WITH THE OTHER EMs
      |
      | CHARGING POWER IS DERIVED FROM THE HP BECAUSE ALL CONFIGURATIONS SHOULD HAVE AN HP EM. IT WILL EFFECTIVELY RAISE THE SUBSYSTEM LOAD.
  note: OUTPUTS
  note: INPUTS
  note: BASE POWER CALCULATION
  note: Standard/Regular
      | Boost
      | Power Extraction
  PwrInLP_Base : Inport
  PwrInHP_Base : Inport  Port=2
  NS : Inport  Port=3
  NR : Inport  Port=4
  NC : Inport  Port=5
  Base Power - Boost and PEx : Subsystem
  Base Power - Standard : Subsystem
  Constant2 : Constant  Value=MWS.In.Options.HybridConfig
  Demux2 : Demux
  Gain : Gain  Gain=-1
  Multiport Switch : MultiPortSwitch
  Multiport Switch1 : MultiPortSwitch
  Subsystem : Subsystem
  Sum of Elements : Sum  Inputs=+
  PwrEMS_Base : Outport
  PwrEMR_Base : Outport  Port=2
  PwrEMC_Base : Outport  Port=3
  PwrEMP_Base : Outport  Port=4
  PwrLoad : Outport  Port=5
  wires:
  PwrInLP_Base/1 -> [PwrL_Base]
  NR/1 -> [NR]
  NS/1 -> [NS]
  NC/1 -> [NC]
  PwrInHP_Base/1 -> [PwrH_Base]
  [PwrEMS_Base] -> PwrEMS_Base/1
  [PwrEMR_Base] -> PwrEMR_Base/1
  [PwrEMC_Base] -> PwrEMC_Base/1
  [PwrEMP_Base] -> PwrEMP_Base/1
  Constant2/1 -> Multiport Switch1/1, Multiport Switch/1
  Multiport Switch/1 -> Demux2/1
  Demux2/1 -> [PwrEMS_Base]
  Demux2/2 -> [PwrEMR_Base]
  Demux2/3 -> [PwrEMC_Base]
  Demux2/4 -> [PwrEMP_Base]
  [PwrH_Base] -> Base Power - Boost and PEx/2(PwrH_Base)
  [NS] -> Base Power - Boost and PEx/3(NS)
  [NR] -> Base Power - Boost and PEx/4(NR)
  [NC] -> Base Power - Boost and PEx/5(NC)
  Base Power - Boost and PEx/1(Pem) -> [Pem_BoostPEx]
  Base Power - Standard/1(Pem) -> [Pem_Std]
  [NC] -> Base Power - Standard/4(NC)
  [NR] -> Base Power - Standard/3(NR)
  [NS] -> Base Power - Standard/2(NS)
  [PwrH_Base] -> Base Power - Standard/1(PwrH_Base)
  [Pem_Std] -> Multiport Switch/2, Multiport Switch1/2, Multiport Switch1/3
  [Pem_BoostPEx] -> Subsystem/1(PwrLoad), Multiport Switch/4, Multiport Switch/3
  [PwrL_Base] -> Base Power - Boost and PEx/1(PwrL_Base)
  Multiport Switch1/1 -> Sum of Elements/1
  Sum of Elements/1 -> Gain/1
  Gain/1 -> [PwrLoad]
  [PwrLoad] -> PwrLoad/1
  Subsystem/1(PwrLoadTot) -> Multiport Switch1/4

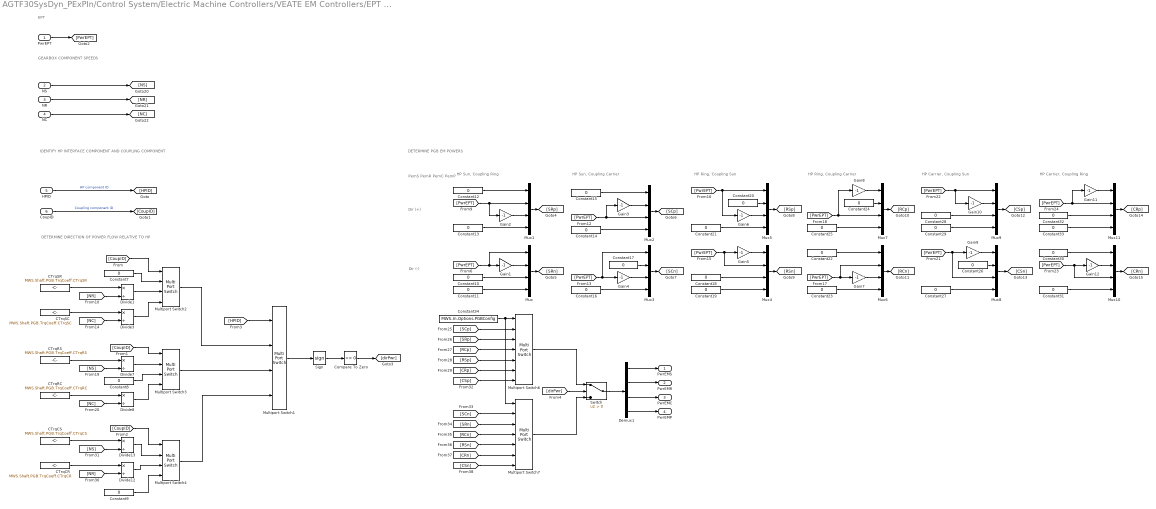
== system AGTF30SysDyn_PExPIn/Control System/Electric Machine Controllers/VEATE EM Controllers/EPT Powers ==
  note: Dir (+)
  note: HP Sun, Coupling Ring
  note: PemS
      | PemR
      | PemC
      | PemP
  note: IDENTIFY HP INTERFACE COMPONENT AND COUPLING COMPONENT
  note: HP Sun, Coupling Carrier
  note: Dir (-)
  note: HP Ring, Coupling Sun
  note: HP Ring, Coupling Carrier
  note: HP Carrier, Coupling Sun
  note: HP Carrier, Coupling Ring
  note: DETERMINE DIRECTION OF POWER FLOW RELATIVE TO HP
  note: DETERMINE PGB EM POWERS
  note: GEARBOX COMPONENT SPEEDS
  note: EPT
  PwrEPT : Inport
  NS : Inport  Port=2
  NR : Inport  Port=3
  NC : Inport  Port=4
  HPID : Inport  Port=5
  CoupID : Inport  Port=6
  CTrqCR : Constant  Value=MWS.Shaft.PGB.TrqCoeff.CTrqCR
  CTrqCS : Constant  Value=MWS.Shaft.PGB.TrqCoeff.CTrqCS
  CTrqRC : Constant  Value=MWS.Shaft.PGB.TrqCoeff.CTrqRC
  CTrqRS : Constant  Value=MWS.Shaft.PGB.TrqCoeff.CTrqRS
  CTrqSC : Constant  Value=MWS.Shaft.PGB.TrqCoeff.CTrqSC
  CTrqSR : Constant  Value=MWS.Shaft.PGB.TrqCoeff.CTrqSR
  Compare To Zero : simulink/Logic and Bit Operations/Compare To Zero  relop=>=  OutDataTypeStr=boolean
  Constant{7..33} (27 alike) : Constant  Value=0
  Constant34 : Constant  Value=MWS.In.Options.PGBConfig
  Demux1 : Demux
  Divide{1,3,7..8,12..13} (6 alike) : Product  Inputs=*/
  Gain{1..12} (12 alike) : Gain  Gain=-1
  Multiport Switch1 : MultiPortSwitch
  Multiport Switch2 : MultiPortSwitch  DataPortOrder=Specify indices
  Multiport Switch3 : MultiPortSwitch  DataPortOrder=Specify indices
  Multiport Switch4 : MultiPortSwitch  DataPortOrder=Specify indices
  Multiport Switch6 : MultiPortSwitch  Inputs=6
  Multiport Switch7 : MultiPortSwitch  Inputs=6
  Mux{,1..11} (12 alike) : Mux
  Sign : Signum
  Switch : Switch  Criteria=u2 > Threshold
  PwrEMS : Outport
  PwrEMR : Outport  Port=2
  PwrEMC : Outport  Port=3
  PwrEMP : Outport  Port=4
  wires:
  HPID/1 -> [HPID]  "HP component ID"
  CoupID/1 -> [CoupID]  "Coupling component ID"
  CTrqSC/1 -> Divide3/1
  [NS] -> Divide13/2
  [NS] -> Divide7/2
  [NC] -> Divide8/2
  [NC] -> Divide3/2
  CTrqCR/1 -> Divide12/1
  [NR] -> Divide12/2
  [NR] -> Divide1/2
  CTrqCS/1 -> Divide13/1
  CTrqRS/1 -> Divide7/1
  CTrqRC/1 -> Divide8/1
  CTrqSR/1 -> Divide1/1
  Divide1/1 -> Multiport Switch2/3
  Divide3/1 -> Multiport Switch2/4
  Constant7/1 -> Multiport Switch2/2
  [CoupID] -> Multiport Switch2/1
  Divide7/1 -> Multiport Switch3/2
  Divide8/1 -> Multiport Switch3/4
  [CoupID] -> Multiport Switch3/1
  Constant8/1 -> Multiport Switch3/3
  Constant9/1 -> Multiport Switch4/4
  [CoupID] -> Multiport Switch4/1
  Divide13/1 -> Multiport Switch4/2
  Divide12/1 -> Multiport Switch4/3
  Multiport Switch3/1 -> Multiport Switch1/3
  Multiport Switch2/1 -> Multiport Switch1/2
  Multiport Switch4/1 -> Multiport Switch1/4
  [HPID] -> Multiport Switch1/1
  Multiport Switch1/1 -> Sign/1
  Sign/1 -> Compare To Zero/1
  Compare To Zero/1 -> [dirPwr]
  Gain1/1 -> Mux/2
  [PwrEPT] -> Mux/1, Gain1/1
  Constant10/1 -> Mux/3
  Constant11/1 -> Mux/4
  Constant13/1 -> Mux1/4
  Constant12/1 -> Mux1/1
  [PwrEPT] -> Mux1/2, Gain2/1
  Gain2/1 -> Mux1/3
  Constant14/1 -> Mux2/4
  [PwrEPT] -> Mux2/3, Gain3/1
  Gain3/1 -> Mux2/2
  Constant15/1 -> Mux2/1
  [PwrEPT] -> Mux3/1, Gain4/1
  Constant16/1 -> Mux3/4
  Gain4/1 -> Mux3/3
  Constant17/1 -> Mux3/2
  [PwrEPT] -> Mux5/1, Gain6/1
  Constant19/1 -> Mux4/4
  [PwrEPT] -> Mux4/2, Gain5/1
  Constant21/1 -> Mux5/4
  Gain6/1 -> Mux5/3
  Gain5/1 -> Mux4/1
  Constant20/1 -> Mux5/2
  Constant18/1 -> Mux4/3
  Constant24/1 -> Mux7/2
  Constant25/1 -> Mux7/4
  [PwrEPT] -> Mux6/2, Gain7/1
  Constant23/1 -> Mux6/4
  [PwrEPT] -> Mux7/3, Gain8/1
  Gain8/1 -> Mux7/1
  Gain7/1 -> Mux6/3
  Constant22/1 -> Mux6/1
  Gain9/1 -> Mux8/1
  Constant27/1 -> Mux8/4
  [PwrEPT] -> Mux8/3, Gain9/1
  Gain10/1 -> Mux9/2
  Constant29/1 -> Mux9/4
  Constant26/1 -> Mux8/2
  [PwrEPT] -> Gain10/1, Mux9/1
  Constant28/1 -> Mux9/3
  Constant32/1 -> Mux11/3
  [PwrEPT] -> Mux11/2, Gain11/1
  Constant33/1 -> Mux11/4
  [PwrEPT] -> Mux10/3, Gain12/1
  Constant31/1 -> Mux10/4
  Gain11/1 -> Mux11/1
  Gain12/1 -> Mux10/2
  Constant30/1 -> Mux10/1
  Mux1/1 -> [SRp]
  Mux/1 -> [SRn]
  Mux2/1 -> [SCp]
  Mux3/1 -> [SCn]
  Mux5/1 -> [RSp]
  Mux4/1 -> [RSn]
  Mux7/1 -> [RCp]
  Mux6/1 -> [RCn]
  Mux9/1 -> [CSp]
  Mux8/1 -> [CSn]
  Mux11/1 -> [CRp]
  Mux10/1 -> [CRn]
  [SCp] -> Multiport Switch6/2
  [SRp] -> Multiport Switch6/3
  [RCp] -> Multiport Switch6/4
  [RSp] -> Multiport Switch6/5
  [CRp] -> Multiport Switch6/6
  [CSp] -> Multiport Switch6/7
  [CSn] -> Multiport Switch7/7
  [CRn] -> Multiport Switch7/6
  [RSn] -> Multiport Switch7/5
  [RCn] -> Multiport Switch7/4
  [SRn] -> Multiport Switch7/3
  [SCn] -> Multiport Switch7/2
  Multiport Switch6/1 -> Switch/1
  Multiport Switch7/1 -> Switch/3
  Switch/1 -> Demux1/1
  Constant34/1 -> Multiport Switch7/1, Multiport Switch6/1
  Demux1/1 -> PwrEMS/1
  Demux1/2 -> PwrEMR/1
  Demux1/3 -> PwrEMC/1
  Demux1/4 -> PwrEMP/1
  PwrEPT/1 -> [PwrEPT]
  NS/1 -> [NS]
  NR/1 -> [NR]
  NC/1 -> [NC]
  [dirPwr] -> Switch/2

== system AGTF30SysDyn_PExPIn/Control System/Electric Machine Controllers/VEATE EM Controllers/TEEM Power ==
  note: TEEM POWER CALCULATION
  note: INPUTS
  note: OUTPUTS
  note: STRATEGY WILL USE THE COUPLING EM AS MUCH AS POSSIBLE AND WILL FILL IN THE REST WITH THE OTHER EMs. OBJECTIVE IS TO ACHIEVE THE DESIRED HP POWER INPUT.
  PwrInHP_TEEM : Inport
  PwrInX_TEEM : Inport  Port=2
  NS : Inport  Port=3
  NR : Inport  Port=4
  NC : Inport  Port=5
  Constant1 : Constant  Value=[0 0 0 0]
  Constant2 : Constant  Value=MWS.In.Options.TEEM
  Demux2 : Demux
  Switch : Switch  Criteria=u2 > Threshold
  TEEM Power : Subsystem
  PwrEMS_TEEM : Outport
  PwrEMR_TEEM : Outport  Port=2
  PwrEMC_TEEM : Outport  Port=3
  PwrEMP_TEEM : Outport  Port=4
  wires:
  TEEM Power/1(Pem) -> [Pem_TEEM]
  [NC] -> TEEM Power/5(NC)
  [NR] -> TEEM Power/4(NR)
  [NS] -> TEEM Power/3(NS)
  [PwrXDecel_TEEM] -> TEEM Power/2(PwrXDecel_TEEM)
  [PwrInAccel_TEEM] -> TEEM Power/1(PwrInAccel_TEEM)
  Demux2/4 -> [PwrEMP_TEEM]
  Demux2/3 -> [PwrEMC_TEEM]
  Demux2/2 -> [PwrEMR_TEEM]
  Demux2/1 -> [PwrEMS_TEEM]
  Constant2/1 -> Switch/2
  [PwrEMP_TEEM] -> PwrEMP_TEEM/1
  [PwrEMC_TEEM] -> PwrEMC_TEEM/1
  [PwrEMR_TEEM] -> PwrEMR_TEEM/1
  [PwrEMS_TEEM] -> PwrEMS_TEEM/1
  PwrInX_TEEM/1 -> [PwrXDecel_TEEM]
  NC/1 -> [NC]
  NS/1 -> [NS]
  NR/1 -> [NR]
  PwrInHP_TEEM/1 -> [PwrInAccel_TEEM]
  [Pem_TEEM] -> Switch/1
  Constant1/1 -> Switch/3
  Switch/1 -> Demux2/1

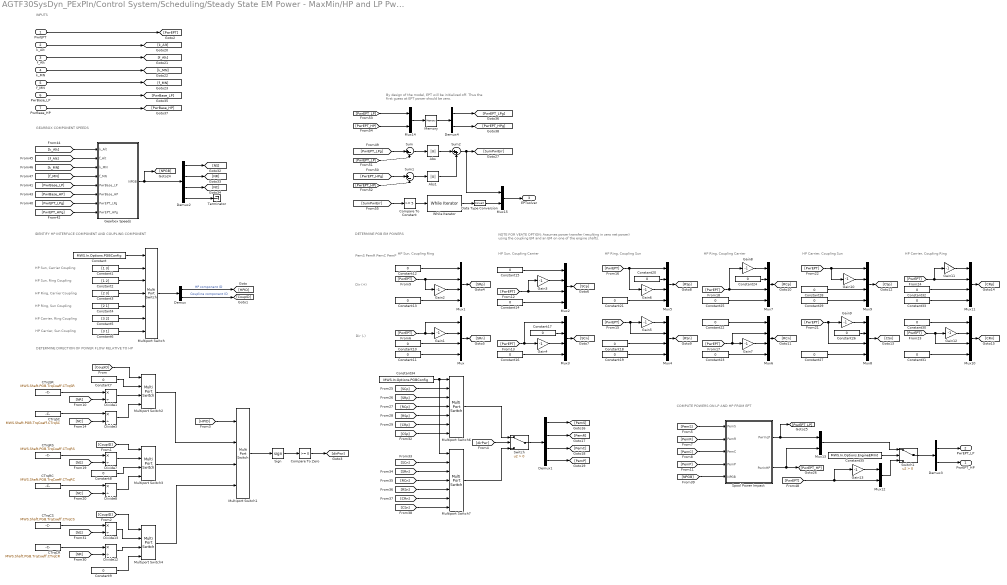
== system AGTF30SysDyn_PExPIn/Control System/Scheduling/Steady State EM Power - MaxMin/HP and LP Pwr Calc ==
  note: By design of the model, EPT will be initialized off. Thus the first guess at EPT power should be zero.
  note: NOTE FOR VEATE OPTION: Assumes power transfer (resulting in zero net power) using the coupling EM and an EM on one of the engine shafts.
  note: Dir (+)
  note: HP Sun, Coupling Ring
  note: PemS
      | PemR
      | PemC
      | PemP
  note: IDENTIFY HP INTERFACE COMPONENT AND COUPLING COMPONENT
  note: HP Sun, Carrier Coupling
  note: HP Sun, Ring Coupling
  note: HP Ring, Carrier Coupling
  note: HP Ring, Sun Coupling
  note: HP Carrier, Ring Coupling
  note: HP Carrier, Sun Coupling
  note: HP Sun, Coupling Carrier
  note: Dir (-)
  note: HP Ring, Coupling Sun
  note: HP Ring, Coupling Carrier
  note: HP Carrier, Coupling Sun
  note: HP Carrier, Coupling Ring
  note: DETERMINE DIRECTION OF POWER FLOW RELATIVE TO HP
  note: DETERMINE PGB EM POWERS
  note: COMPUTE POWERS ON LP AND HP FROM EPT
  note: GEARBOX COMPONENT SPEEDS
  note: INPUTS
  PwrEPT : Inport
  k_Alt : Inport  Port=2
  f_Alt : Inport  Port=3
  k_MN : Inport  Port=4
  f_MN : Inport  Port=5
  PwrBase_LP : Inport  Port=6
  PwrBase_HP : Inport  Port=7
  Abs : Abs
  Abs1 : Abs
  CTrqCR : Constant  Value=MWS.Shaft.PGB.TrqCoeff.CTrqCR
  CTrqCS : Constant  Value=MWS.Shaft.PGB.TrqCoeff.CTrqCS
  CTrqRC : Constant  Value=MWS.Shaft.PGB.TrqCoeff.CTrqRC
  CTrqRS : Constant  Value=MWS.Shaft.PGB.TrqCoeff.CTrqRS
  CTrqSC : Constant  Value=MWS.Shaft.PGB.TrqCoeff.CTrqSC
  CTrqSR : Constant  Value=MWS.Shaft.PGB.TrqCoeff.CTrqSR
  Compare To Constant : simulink/Logic and Bit Operations/Compare To Constant  relop=>=  const=5  OutDataTypeStr=boolean
  Compare To Zero : simulink/Logic and Bit Operations/Compare To Zero  relop=>=  OutDataTypeStr=boolean
  Constant : Constant  Value=MWS.In.Options.PGBConfig
  Constant1 : Constant  Value=[1 3]
  Constant{7..33} (27 alike) : Constant  Value=0
  Constant2 : Constant  Value=[1 2]
  Constant3 : Constant  Value=[2 3]
  Constant34 : Constant  Value=MWS.In.Options.PGBConfig
  Constant35 : Constant  Value=MWS.In.Options.EngineEMInt
  Constant4 : Constant  Value=[2 1]
  Constant5 : Constant  Value=[3 2]
  Constant6 : Constant  Value=[3 1]
  Data Type Conversion : DataTypeConversion
  Demux : Demux  Outputs=2
  Demux1 : Demux
  Demux2 : Demux
  Demux3 : Demux  Outputs=2
  Demux4 : Demux  Outputs=2
  Divide{1,3,7..8,12..13} (6 alike) : Product  Inputs=*/
  Gain{1..13} (13 alike) : Gain  Gain=-1
  Gearbox Speeds : Subsystem
  Memory : Memory  InitialCondition=[0 0]  InheritSampleTime=on
  Multiport Switch : MultiPortSwitch  Inputs=6
  Multiport Switch1 : MultiPortSwitch
  Multiport Switch2 : MultiPortSwitch  DataPortOrder=Specify indices
  Multiport Switch3 : MultiPortSwitch  DataPortOrder=Specify indices
  Multiport Switch4 : MultiPortSwitch  DataPortOrder=Specify indices
  Multiport Switch6 : MultiPortSwitch  Inputs=6
  Multiport Switch7 : MultiPortSwitch  Inputs=6
  Mux{,1..11} (12 alike) : Mux
  Mux{12..15} (4 alike) : Mux  Inputs=2
  Sign : Signum
  Spool Power Impact : Subsystem
  Sum : Sum  Inputs=|+-
  Sum1 : Sum  Inputs=|+-
  Sum2 : Sum  Inputs=|++
  Switch : Switch  Criteria=u2 > Threshold
  Switch1 : Switch  Criteria=u2 > Threshold
  Terminator : Terminator
  While Iterator : WhileIterator  MaxIters=10  WhileBlockType=do-while  ShowIterationPort=on
  PwrEPT_HP : Outport
  PwrEPT_LP : Outport  Port=2
  EPTsolver : Outport  Port=3
  wires:
  Constant/1 -> Multiport Switch/1
  Constant2/1 -> Multiport Switch/3
  Constant1/1 -> Multiport Switch/2
  Constant3/1 -> Multiport Switch/4
  Constant4/1 -> Multiport Switch/5
  Constant5/1 -> Multiport Switch/6
  Constant6/1 -> Multiport Switch/7
  Multiport Switch/1 -> Demux/1
  Demux/1 -> [HPID]  "HP component ID"
  Demux/2 -> [CoupID]  "Coupline component ID"
  CTrqSC/1 -> Divide3/1
  [NS] -> Divide13/2
  [NS] -> Divide7/2
  [NC] -> Divide8/2
  [NC] -> Divide3/2
  CTrqCR/1 -> Divide12/1
  [NR] -> Divide12/2
  [NR] -> Divide1/2
  CTrqCS/1 -> Divide13/1
  CTrqRS/1 -> Divide7/1
  CTrqRC/1 -> Divide8/1
  CTrqSR/1 -> Divide1/1
  Divide1/1 -> Multiport Switch2/3
  Divide3/1 -> Multiport Switch2/4
  Constant7/1 -> Multiport Switch2/2
  [CoupID] -> Multiport Switch2/1
  Divide7/1 -> Multiport Switch3/2
  Divide8/1 -> Multiport Switch3/4
  [CoupID] -> Multiport Switch3/1
  Constant8/1 -> Multiport Switch3/3
  Constant9/1 -> Multiport Switch4/4
  [CoupID] -> Multiport Switch4/1
  Divide13/1 -> Multiport Switch4/2
  Divide12/1 -> Multiport Switch4/3
  Multiport Switch3/1 -> Multiport Switch1/3
  Multiport Switch2/1 -> Multiport Switch1/2
  Multiport Switch4/1 -> Multiport Switch1/4
  [HPID] -> Multiport Switch1/1
  Multiport Switch1/1 -> Sign/1
  Sign/1 -> Compare To Zero/1
  Compare To Zero/1 -> [dirPwr]
  [dirPwr] -> Switch/2
  Gain1/1 -> Mux/2
  [PwrEPT] -> Mux/1, Gain1/1
  Constant10/1 -> Mux/3
  Constant11/1 -> Mux/4
  Constant13/1 -> Mux1/4
  Constant12/1 -> Mux1/1
  [PwrEPT] -> Mux1/2, Gain2/1
  Gain2/1 -> Mux1/3
  Constant14/1 -> Mux2/4
  [PwrEPT] -> Mux2/3, Gain3/1
  Gain3/1 -> Mux2/2
  Constant15/1 -> Mux2/1
  [PwrEPT] -> Mux3/1, Gain4/1
  Constant16/1 -> Mux3/4
  Gain4/1 -> Mux3/3
  Constant17/1 -> Mux3/2
  [PwrEPT] -> Mux5/1, Gain6/1
  Constant19/1 -> Mux4/4
  [PwrEPT] -> Mux4/2, Gain5/1
  Constant21/1 -> Mux5/4
  Gain6/1 -> Mux5/3
  Gain5/1 -> Mux4/1
  Constant20/1 -> Mux5/2
  Constant18/1 -> Mux4/3
  Constant24/1 -> Mux7/2
  Constant25/1 -> Mux7/4
  [PwrEPT] -> Mux6/2, Gain7/1
  Constant23/1 -> Mux6/4
  [PwrEPT] -> Mux7/3, Gain8/1
  Gain8/1 -> Mux7/1
  Gain7/1 -> Mux6/3
  Constant22/1 -> Mux6/1
  Gain9/1 -> Mux8/1
  Constant27/1 -> Mux8/4
  [PwrEPT] -> Mux8/3, Gain9/1
  Gain10/1 -> Mux9/2
  Constant29/1 -> Mux9/4
  Constant26/1 -> Mux8/2
  [PwrEPT] -> Gain10/1, Mux9/1
  Constant28/1 -> Mux9/3
  Constant32/1 -> Mux11/3
  [PwrEPT] -> Mux11/2, Gain11/1
  Constant33/1 -> Mux11/4
  [PwrEPT] -> Mux10/3, Gain12/1
  Constant31/1 -> Mux10/4
  Gain11/1 -> Mux11/1
  Gain12/1 -> Mux10/2
  Constant30/1 -> Mux10/1
  Mux1/1 -> [SRp]
  Mux/1 -> [SRn]
  Mux2/1 -> [SCp]
  Mux3/1 -> [SCn]
  Mux5/1 -> [RSp]
  Mux4/1 -> [RSn]
  Mux7/1 -> [RCp]
  Mux6/1 -> [RCn]
  Mux9/1 -> [CSp]
  Mux8/1 -> [CSn]
  Mux11/1 -> [CRp]
  Mux10/1 -> [CRn]
  [SCp] -> Multiport Switch6/2
  [SRp] -> Multiport Switch6/3
  [RCp] -> Multiport Switch6/4
  [RSp] -> Multiport Switch6/5
  [CRp] -> Multiport Switch6/6
  [CSp] -> Multiport Switch6/7
  [CSn] -> Multiport Switch7/7
  [CRn] -> Multiport Switch7/6
  [RSn] -> Multiport Switch7/5
  [RCn] -> Multiport Switch7/4
  [SRn] -> Multiport Switch7/3
  [SCn] -> Multiport Switch7/2
  Multiport Switch6/1 -> Switch/1
  Multiport Switch7/1 -> Switch/3
  Switch/1 -> Demux1/1
  Constant34/1 -> Multiport Switch7/1, Multiport Switch6/1
  Demux1/1 -> [PemS]
  Demux1/2 -> [PemR]
  Demux1/3 -> [PemC]
  Demux1/4 -> [PemP]
  [PemS] -> Spool Power Impact/1(PemS)
  [PemR] -> Spool Power Impact/2(PemR)
  [PemC] -> Spool Power Impact/3(PemC)
  [PemP] -> Spool Power Impact/4(PemP)
  [k_Alt] -> Gearbox Speeds/1(k_Alt)
  [f_Alt] -> Gearbox Speeds/2(f_Alt)
  [k_MN] -> Gearbox Speeds/3(k_MN)
  [f_MN] -> Gearbox Speeds/4(f_MN)
  [PwrBase_LP] -> Gearbox Speeds/5(PwrBase_LP)
  [PwrEPT_LPg] -> Gearbox Speeds/7(PwrEPT_LPg)
  [PwrBase_HP] -> Gearbox Speeds/6(PwrBase_HP)
  [PwrEPT_HPg] -> Gearbox Speeds/8(PwrEPT_HPg)
  Gearbox Speeds/1(NPGB) -> Demux2/1, [NPGB]
  Demux2/1 -> [NS]
  Demux2/3 -> [NC]
  Demux2/2 -> [NR]
  Demux2/4 -> Terminator/1
  [NPGB] -> Spool Power Impact/5(NPGB)
  k_Alt/1 -> [k_Alt]
  f_Alt/1 -> [f_Alt]
  k_MN/1 -> [k_MN]
  f_MN/1 -> [f_MN]
  PwrBase_LP/1 -> [PwrBase_LP]
  PwrBase_HP/1 -> [PwrBase_HP]
  [PwrEPT] -> Mux12/2, Gain13/1
  Switch1/1 -> Demux3/1
  Mux13/1 -> Switch1/1
  Mux12/1 -> Switch1/3
  Constant35/1 -> Switch1/2
  Demux3/2 -> PwrEPT_HP/1
  Demux3/1 -> PwrEPT_LP/1
  Spool Power Impact/1(PwrInLP) -> [PwrEPT_LP], Mux13/1
  Spool Power Impact/2(PwrInHP) -> Mux13/2, [PwrEPT_HP]
  PwrEPT/1 -> [PwrEPT]
  [PwrEPT_LPg] -> Sum/1
  [PwrEPT_LP] -> Sum/2
  [PwrEPT_HPg] -> Sum1/1
  [PwrEPT_HP] -> Sum1/2
  Sum/1 -> Abs/1
  Sum1/1 -> Abs1/1
  Abs/1 -> Sum2/1
  Abs1/1 -> Sum2/2
  Sum2/1 -> Mux15/1, [SumPwrErr]
  Memory/1 -> Demux4/1
  Demux4/1 -> [PwrEPT_LPg]
  Demux4/2 -> [PwrEPT_HPg]
  Mux14/1 -> Memory/1
  [PwrEPT_LP] -> Mux14/1
  [PwrEPT_HP] -> Mux14/2
  Compare To Constant/1 -> While Iterator/1
  [SumPwrErr] -> Compare To Constant/1
  While Iterator/1 -> Data Type Conversion/1
  Mux15/1 -> EPTsolver/1
  Data Type Conversion/1 -> Mux15/2
  Gain13/1 -> Mux12/1
